simulink model "SistemaCAS_v7"  (R2014a)
settings: Solver=ode45  StartTime=0.0  StopTime=100.0  RelTol=1e-3
settings Model: Creator=andre  LastModifiedBy=andre

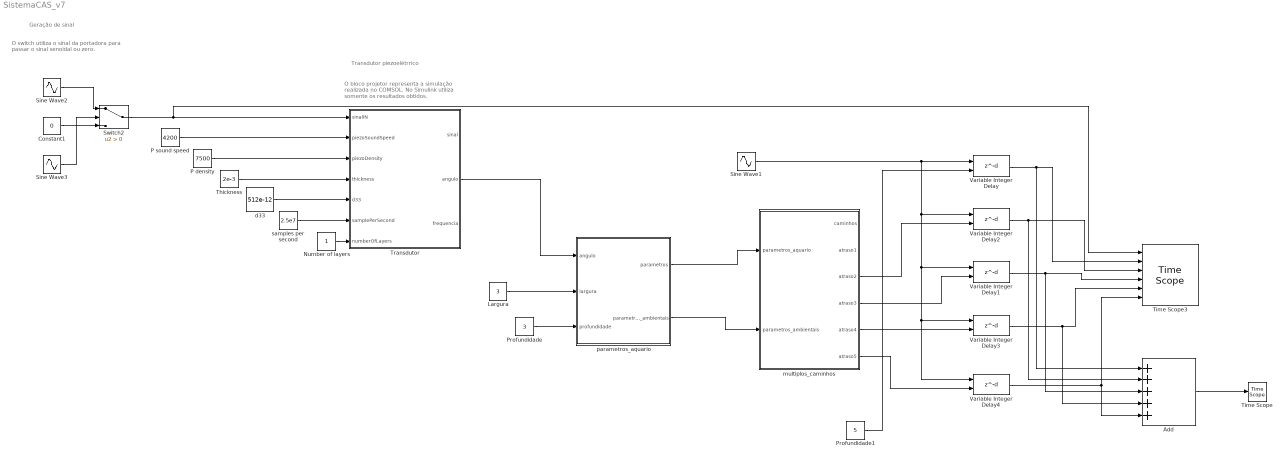
== system SistemaCAS_v7 ==
  note: Geração de sinal
  note: O bloco projetor representa a simulação
      | realizada no COMSOL. No Simulink utiliza
      | somente os resultados obtidos.
  note: O switch utiliza o sinal da portadora
      | para passar o sinal senoidal ou zero.
  note: Transdutor piezoelétrrico
  Add : Sum  Inputs=+++++
  Constant1 : Constant  Value=0
  Largura : Constant  Value=3
  Number of layers : Constant
  P density : Constant  Value=7500
  P sound speed : Constant  Value=4200
  Profundidade : Constant  Value=3
  Profundidade1 : Constant  Value=5
  Sine Wave1 : Sin  Frequency=5  SampleTime=1
  Sine Wave2 : Sin  Frequency=5  SampleTime=0
  Sine Wave3 : Sin  SampleTime=0
  Switch2 : Switch  Criteria=u2 > Threshold
  Thickness : Constant  Value=2e-3
  Time Scope : TimeScope  DefaultConfigurationName=spbscopes.TimeScopeBlockCfg
  Time Scope3 : TimeScope  NumInputPorts=6  DefaultConfigurationName=spbscopes.TimeScopeBlockCfg
  Transdutor : MATLAB Function  TreatAsAtomicUnit=on
  Variable Integer Delay{,1..4} (5 alike) : Delay  DelayLengthSource=Input port
      settings: InputPortMap=u0,p1
  d33 : Constant  Value=512e-12
  multiplos_caminhos : MATLAB Function  TreatAsAtomicUnit=on
  parametros_aquario : MATLAB Function  TreatAsAtomicUnit=on
  samples per second : Constant  Value=2.5e7
  wires:
  d33/1 -> Transdutor/5(d33)
  samples per second/1 -> Transdutor/6(samplePerSecond)
  Number of layers/1 -> Transdutor/7(numberOfLayers)
  P sound speed/1 -> Transdutor/2(piezoSoundSpeed)
  P density/1 -> Transdutor/3(piezoDensity)
  Thickness/1 -> Transdutor/4(thickness)
  Largura/1 -> parametros_aquario/2(largura)
  Profundidade/1 -> parametros_aquario/3(profundidade)
  Transdutor/2(angulo) -> parametros_aquario/1(angulo)
  parametros_aquario/1(parametros) -> multiplos_caminhos/1(parametros_aquario)
  Sine Wave1/1 -> Variable Integer Delay4/1, Variable Integer Delay3/1, Variable Integer Delay1/1, Variable Integer Delay2/1, Variable Integer Delay/1
  parametros_aquario/2(parametros_ambientais) -> multiplos_caminhos/2(parametros_ambientais)
  Sine Wave2/1 -> Switch2/1
  Sine Wave3/1 -> Switch2/2
  Constant1/1 -> Switch2/3
  Switch2/1 -> Time Scope3/1, Transdutor/1(sinalIN)
  Profundidade1/1 -> Variable Integer Delay/2
  multiplos_caminhos/3(atraso2) -> Variable Integer Delay2/2
  multiplos_caminhos/4(atraso3) -> Variable Integer Delay1/2
  multiplos_caminhos/5(atraso4) -> Variable Integer Delay3/2
  multiplos_caminhos/6(atraso5) -> Variable Integer Delay4/2
  Variable Integer Delay1/1 -> Add/3, Time Scope3/4
  Variable Integer Delay3/1 -> Add/4, Time Scope3/5
  Variable Integer Delay2/1 -> Add/2, Time Scope3/3
  Variable Integer Delay/1 -> Add/1, Time Scope3/2
  Variable Integer Delay4/1 -> Time Scope3/6, Add/5
  Add/1 -> Time Scope/1

== matlab function SistemaCAS_v7/parametros_aquario ==
  data: angulo input; largura input; profundidade input; parametros output; parametros_ambientais output
function [parametros,parametros_ambientais] = parametros_aquario(angulo,largura,profundidade)
% consideraçoes para os parâmetros do aquário
% 1. emissor e receptor estão alinhados ( largura(x) e profundidade(z)
% iguais, só muda o comprimento (y)
% 2. o comprimento do aquario (L) é ideal para acontecer uma reflexão completa
% com o angulo de diretividade (que é o maior angulo possível do lóbulo 
% principal utilizando o transdutor piezoeletrico escolhido)
% 3. para facilitar os cálculos de do comprimento ideal, utilizamos largura
% igual profundidade (D = W)

% considerações sobre a simulação
% 1. serão considerados somente os caminhos do angulo de diretividade e o
% caminho direto (5 caminhos: um direto, dois que refletem nas laterais, e
% dois que refletem na superfície e o fundo
% 2. a reflexão será considerada reflexão completa com um eco (sem perdas 
% de energia ou refraçao)

%-------------------------------------------------------------------------
%Parâmetros do Aquário definidos anteriormente
%-------------------------------------------------------------------------
w = largura;                  % largura (eixo x)
d = profundidade;             % profundidade do aquário (eixo z) 
l = w/sin(angulo/2);      % comprimento do aquário calculado utilizando o angulo de diretividade (eixo y)
% l(éle) é a distancia ideal para acontecer uma reflexão completa
parametros = [w,l,d];


%-------------------------------------------------------------------------
% Valores dos parâmetros do meio subaquático 
%-------------------------------------------------------------------------
T = 32;                 % Temperatura (°C)
S = 1;                  % Salinidade (ppt)
pH = 7.2;               % acidêz da água - pH (potencial hidrogeniônico)
parametros_ambientais = [T, S, pH];

== matlab function SistemaCAS_v7/multiplos_caminhos ==
  data: caminhos output; atraso1 output; atraso2 output; atraso3 output; atraso4 output; atraso5 output; parametros_aquario input; parametros_ambientais input
function [caminhos,atraso1,atraso2,atraso3,atraso4,atraso5] = multiplos_caminhos(parametros_aquario,parametros_ambientais)
%Definir as distâncias de cada caminho
%Atrasar o sinal de cada caminho
%Enviar a distância e o sinal de cada caminho ()

w = parametros_aquario(1);
l = parametros_aquario(2);
d = parametros_aquario(3);

T = parametros_ambientais(1);
S = parametros_ambientais(2);
pH = parametros_ambientais(3);

%%%%%%  Bloco multipath  %%%%%%

%-------------------------------------------------------------------------
%Definindo as distâncias de cada caminho do multipath
%-------------------------------------------------------------------------
% caminho_1 = caminho refletido na superfície
% caminho_2 = caminho refletido na lateral de trás
% caminho_3 = caminho direto
% caminho_4 = caminho refletido na lateral da frente
% caminho_5 = caminho refletido no fundo
caminhos = [0 0 0 0 0];
caminhos(1) = sqrt(d^2 + l^2);
caminhos(2) = sqrt(w^2 + l^2);
caminhos(3) = l;
caminhos(4) = caminhos(2);
caminhos(5) = caminhos(1);

%-------------------------------------------------------------------------
%Definindo a profundidade média para cada caminho
%-------------------------------------------------------------------------
D = [0 0 0 0 0];
D(1) = mean([d/2,0]);
D(2) = d/2;
D(3) = d/2;
D(4) = d/2;
D(5) = mean([d,d/2]);

%-------------------------------------------------------------------------
%Velocidade do som na água (m/s)
%-------------------------------------------------------------------------
C = [0 0 0 0 0];
for i = 1:5 %5 caminhos
    c = 1448.96 + 4.591*T - 5.304*(10^(-2))*(T^(2))...
        + 2.374*(10^(-4))*(T^(3)) + 1.340*(S-35) + 1.630*(10^(-2))*D(i)...
        + 1.675*(10^(-7))*(D(i)^(2)) - 1.025*(10^(-2))*T*(S-35)...
        - 7.139*(10^(-13))*T*(D(i)^(3));
    
    %Conversão de (m/s) para (cm/s)
    C(i)=c*100;
end

%-------------------------------------------------------------------------
% Definindo os atrasos de cada caminho do multipath através da equação de
% velocidade de propagação do som na água
%-------------------------------------------------------------------------

% atraso é o tempo que o caminho leva

atraso1 = D(1)/C(1);
atraso2 = D(2)/C(2);
atraso3 = D(3)/C(3); % caminho direto não tem atraso
atraso4 = D(4)/C(4);
atraso5 = D(5)/C(5);

== matlab function SistemaCAS_v7/Transdutor ==
  data: sinalIN input; sinal output; piezoSoundSpeed input; piezoDensity input; thickness input; d33 input; samplePerSecond input; numberOfLayers input; angulo output; frequencia output
function [sinal, angulo, frequencia] = projetor(sinalIN, piezoSoundSpeed, piezoDensity, thickness, d33, samplePerSecond, numberOfLayers)


%-------------------------------------------------------------------------
% Sinal 
%-------------------------------------------------------------------------
sinal=sinalIN;

%-------------------------------------------------------------------------
% Ângulo de diretividade do transdutor calculado no COMSOL (rad)
%-------------------------------------------------------------------------
angulo = pi/3;            % (ex.: 60º = pi/3 rad)

%-------------------------------------------------------------------------
% Frequência do Sinal (kHz)
%-------------------------------------------------------------------------
frequencia = 1:2:2000;
